simulink subsystem "NoThermalEffect"  (R2025b)
settings: Solver=VariableStepAuto  StartTime=0.0  StopTime=10.0  RelTol=1e-3
undefined symbols (not defined in the file): Qbatt, Qem, Qpwre
settings Model: ModifiedByFormat=The MathWorks, Inc.  Creator=The MathWorks, Inc.  LastModifiedBy=The MathWorks, Inc.
settings RTWCC: GPUComputeCapability=3.5

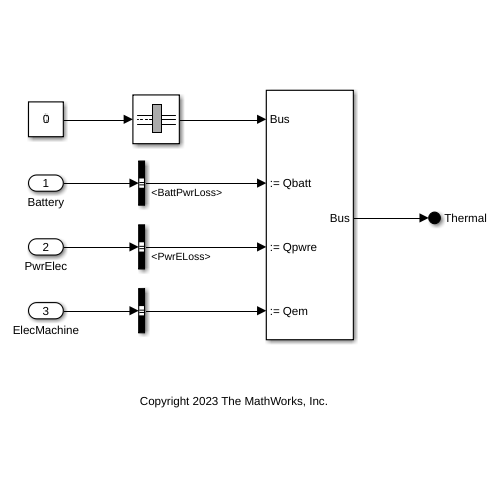
[thumbnail: Simulink's stored preview of the top-level diagram]
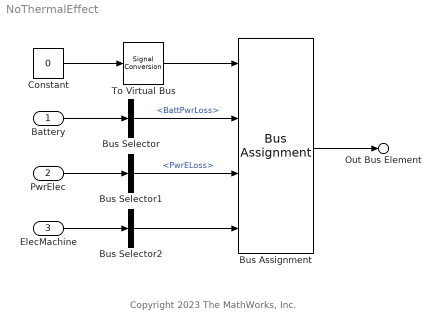
== system NoThermalEffect ==
  note: Copyright 2023 The MathWorks, Inc.
  Battery : Inport
  PwrElec : Inport  Port=2
  ElecMachine : Inport  Port=3
  Bus Assignment : BusAssignment  AssignedSignals=Qbatt,Qpwre,Qem
  Bus Selector : BusSelector  OutputSignals=BattInfo.BattPwrLoss
  Bus Selector1 : BusSelector  OutputSignals=PwrELoss
  Bus Selector2 : BusSelector  OutputSignals=EMPwrLoss  OutputAsBus=on
  Constant : Constant  Value=0  OutDataTypeStr=Bus: ThermalBUS  SampleTime=-1
  To Virtual Bus : SignalConversion  ConversionOutput=Virtual bus  OverrideOpt=off
  Out Bus Element : Outport  PortName=Thermal
  wires:
  Bus Assignment/1 -> Out Bus Element/1
  Bus Selector2/1 -> Bus Assignment/4
  Bus Selector/1 -> Bus Assignment/2  "<BattPwrLoss>"
  Battery/1 -> Bus Selector/1
  PwrElec/1 -> Bus Selector1/1
  Bus Selector1/1 -> Bus Assignment/3  "<PwrELoss>"
  ElecMachine/1 -> Bus Selector2/1
  To Virtual Bus/1 -> Bus Assignment/1
  Constant/1 -> To Virtual Bus/1
